simulink model "hierarchical"  (Simulink 7.2)
settings: Solver=FixedStepDiscrete  StartTime=0.0  StopTime=10.0  FixedStep=1.0  RelTol=1e-3
values from neighbouring files (symbols this model uses):
  IC = 0.6    [constants.mat]
settings Model: Creator=arnaud  LastModifiedBy=arnaud

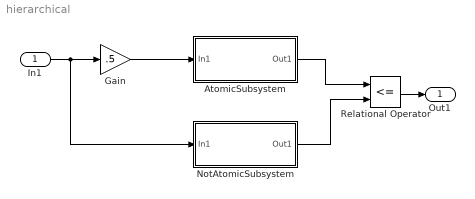
== system hierarchical ==
  In1 : Inport
  AtomicSubsystem : Subsystem  TreatAsAtomicUnit=on
  Gain : Gain  Gain=.5  ParameterDataType=sfix(16)  ParameterScaling=2^0  OutDataType=sfix(16)  OutScaling=2^0
  NotAtomicSubsystem : Subsystem
  Relational Operator : RelationalOperator  Operator=<=  LogicOutDataTypeMode=boolean  OutDataTypeStr=boolean
  Out1 : Outport
  wires:
  In1/1 -> Gain/1, NotAtomicSubsystem/1(In1)
  Gain/1 -> AtomicSubsystem/1(In1)
  AtomicSubsystem/1(Out1) -> Relational Operator/1
  NotAtomicSubsystem/1(Out1) -> Relational Operator/2
  Relational Operator/1 -> Out1/1

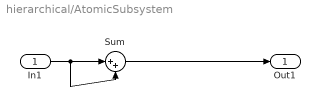
== system hierarchical/AtomicSubsystem ==
  In1 : Inport  OutDataType=sfix(16)  OutScaling=2^0
  Sum : Sum  Inputs=|++  OutDataType=sfix(16)  OutScaling=2^0
  Out1 : Outport  OutDataType=sfix(16)  OutScaling=2^0
  wires:
  In1/1 -> Sum/1, Sum/2
  Sum/1 -> Out1/1

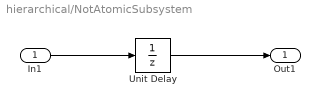
== system hierarchical/NotAtomicSubsystem ==
  In1 : Inport  OutDataType=sfix(16)  OutScaling=2^0
  Unit Delay : UnitDelay  X0=IC
  Out1 : Outport  OutDataType=sfix(16)  OutScaling=2^0
  wires:
  In1/1 -> Unit Delay/1
  Unit Delay/1 -> Out1/1
